simulink model "test_model_ver1"  (R2018a)
settings: Solver=FixedStepAuto  StartTime=0.0  StopTime=789  FixedStep=1  RelTol=1e-3
PreLoadFcn:
  | load '../simulink/model_specs/LSTM/n_LSTM_units.mat'
  | load '../simulink/model_specs/LSTM/T.mat'
  | load '../simulink/model_specs/LSTM/data_input_weights.mat'
  | load '../simulink/model_specs/LSTM/h_weights.mat'
  | load '../simulink/model_specs/LSTM/gate_bias.mat'
  | load '../simulink/model_specs/MLP/weight1.mat'
  | load '../simulink/model_specs/MLP/bias1.mat'
  | load '../simulink/model_specs/MLP/weight2.mat'
  | load '../simulink/model_specs/MLP/bias2.mat'
PostLoadFcn:
  | load 'model_specs/LSTM/n_LSTM_units.mat'
  | load 'model_specs/LSTM/T.mat'
  | load 'model_specs/LSTM/data_input_weights.mat'
  | load 'model_specs/LSTM/h_weights.mat'
  | load 'model_specs/LSTM/gate_bias.mat'
  | load 'model_specs/MLP/weight1.mat'
  | load 'model_specs/MLP/bias1.mat'
  | load 'model_specs/MLP/weight2.mat'
  | load 'model_specs/MLP/bias2.mat'
undefined symbols (not defined in the file): bias1, bias2, data_input_weights, gate_bias, h_weights, n_LSTM_units, weight1, weight2
settings Model: Creator=tongl  LastModifiedBy=tongl

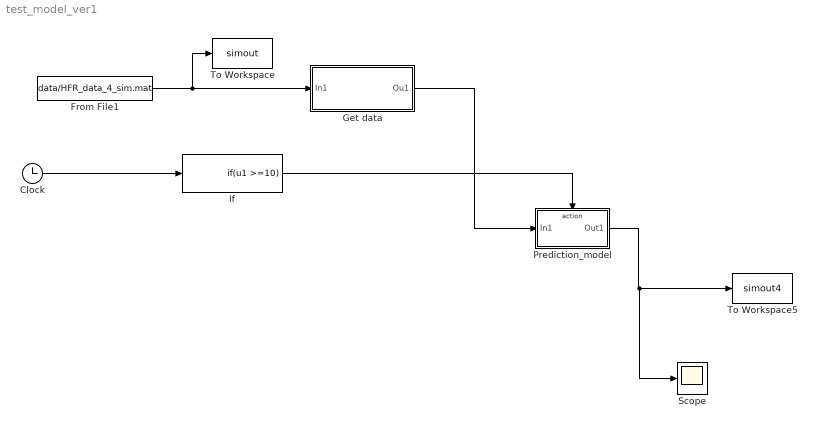
== system test_model_ver1 ==
  Clock : Clock
  From File1 : FromFile  FileName=data/HFR_data_4_sim.mat  OutDataTypeStr=double  SampleTime=1  ExtrapolationBeforeFirstDataPoint=Hold first value
  Get data : Subsystem  Tag=Get_Data
  If : If  IfExpression=u1 >=10  ShowElse=off
  "Prediction_model " : Subsystem  TreatAsAtomicUnit=on
  Scope : Scope
  To Workspace : ToWorkspace  VariableName=simout  SaveFormat=Timeseries  SampleTime=-1
  To Workspace5 : ToWorkspace  VariableName=simout4  SaveFormat=Timeseries  SampleTime=-1
  wires:
  Clock/1 -> If/1
  If/1 -> "Prediction_model "/Action
  "Prediction_model "/1(Out1) -> Scope/1, To Workspace5/1
  From File1/1 -> To Workspace/1, Get data/1(In1)
  Get data/1(Ou1) -> "Prediction_model "/1(In1)

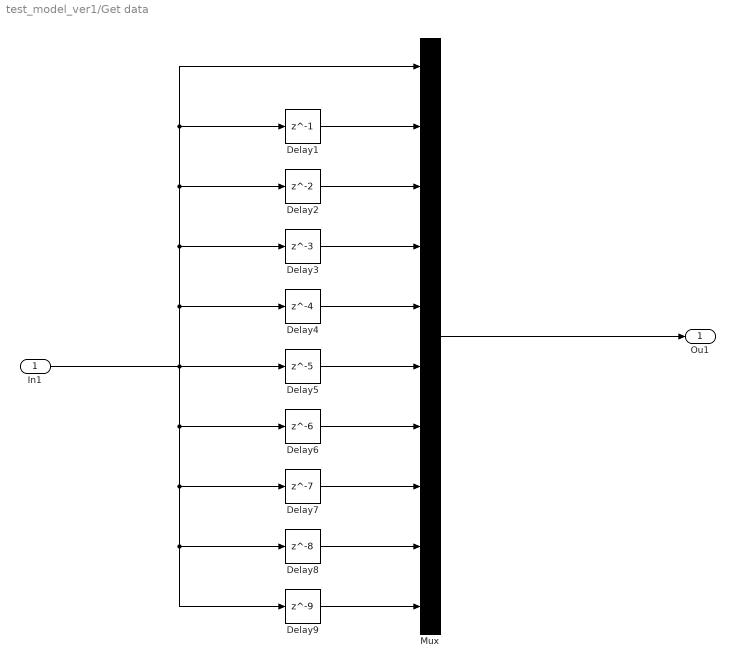
== system test_model_ver1/Get data ==
  In1 : Inport
  Delay1 : Delay  DelayLength=1  InitialCondition=0
  Delay2 : Delay  InitialCondition=0
  Delay3 : Delay  DelayLength=3  InitialCondition=0
  Delay4 : Delay  DelayLength=4  InitialCondition=0
  Delay5 : Delay  DelayLength=5  InitialCondition=0
  Delay6 : Delay  DelayLength=6  InitialCondition=0
  Delay7 : Delay  DelayLength=7  InitialCondition=0
  Delay8 : Delay  DelayLength=8  InitialCondition=0
  Delay9 : Delay  DelayLength=9  InitialCondition=0
  Mux : Mux  Inputs=10
  Ou1 : Outport
  wires:
  Delay2/1 -> Mux/3
  Delay3/1 -> Mux/4
  Delay8/1 -> Mux/9
  Delay7/1 -> Mux/8
  Delay6/1 -> Mux/7
  Delay4/1 -> Mux/5
  Delay1/1 -> Mux/2
  Delay9/1 -> Mux/10
  Delay5/1 -> Mux/6
  Mux/1 -> Ou1/1
  In1/1 -> Delay7/1, Delay9/1, Delay8/1, Delay6/1, Delay5/1, Delay4/1, Delay3/1, Delay2/1, Mux/1, Delay1/1

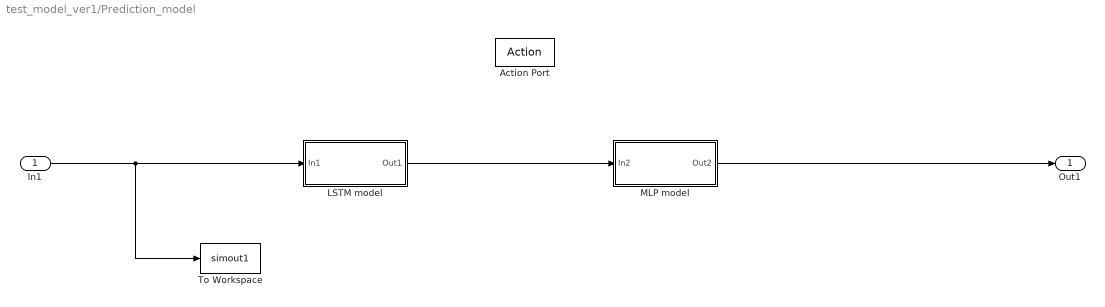
== system test_model_ver1/Prediction_model  ==
  In1 : Inport
  Action Port : ActionPort  ActionType=then
  LSTM model : Subsystem  TreatAsAtomicUnit=on
  MLP model : Subsystem
  To Workspace : ToWorkspace  VariableName=simout1  SaveFormat=Timeseries  SampleTime=-1
  Out1 : Outport
  wires:
  In1/1 -> To Workspace/1, LSTM model/1(In1)
  LSTM model/1(Out1) -> MLP model/1(In2)
  MLP model/1(Out2) -> Out1/1

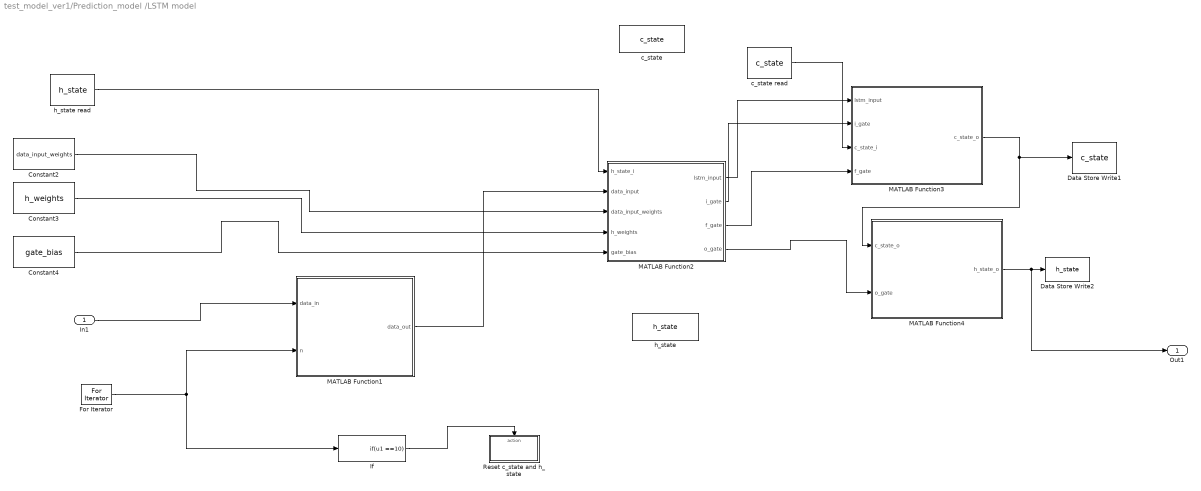
== system test_model_ver1/Prediction_model /LSTM model ==
  In1 : Inport
  Constant2 : Constant  Value=data_input_weights
  Constant3 : Constant  Value=h_weights
  Constant4 : Constant  Value=gate_bias
  Data Store Write1 : DataStoreWrite  DataStoreName=c_state
  Data Store Write2 : DataStoreWrite  DataStoreName=h_state
  For Iterator : ForIterator  IterationLimit=10
  If : If  IfExpression=u1 ==10  ShowElse=off
  MATLAB Function1 : MATLAB Function  TreatAsAtomicUnit=on
  MATLAB Function2 : MATLAB Function  TreatAsAtomicUnit=on
  MATLAB Function3 : MATLAB Function  TreatAsAtomicUnit=on
  MATLAB Function4 : MATLAB Function  TreatAsAtomicUnit=on
  Reset c_state and h_state : Subsystem  TreatAsAtomicUnit=on
  c_state : DataStoreMemory  DataStoreName=c_state  ReadBeforeWriteMsg=warning  WriteAfterWriteMsg=warning  WriteAfterReadMsg=warning  InitialValue=zeros(256,1)  ShowAdditionalParam=off  OutDataTypeStr=single  Dimensions=[n_LSTM_units,1]
  c_state read : DataStoreRead  DataStoreName=c_state
  h_state : DataStoreMemory  DataStoreName=h_state  ReadBeforeWriteMsg=warning  WriteAfterWriteMsg=warning  WriteAfterReadMsg=warning  InitialValue=zeros(256,1)  ShowAdditionalParam=off  OutDataTypeStr=single  Dimensions=[n_LSTM_units,1]
  h_state read : DataStoreRead  DataStoreName=h_state
  Out1 : Outport
  wires:
  h_state read/1 -> MATLAB Function2/1(h_state_i)
  MATLAB Function4/1(h_state_o) -> Out1/1, Data Store Write2/1
  Constant3/1 -> MATLAB Function2/4(h_weights)
  MATLAB Function3/1(c_state_o) -> MATLAB Function4/1(c_state_o), Data Store Write1/1
  MATLAB Function2/4(o_gate) -> MATLAB Function4/2(o_gate)
  MATLAB Function2/1(lstm_input) -> MATLAB Function3/1(lstm_input)
  Constant2/1 -> MATLAB Function2/3(data_input_weights)
  c_state read/1 -> MATLAB Function3/3(c_state_i)
  MATLAB Function2/2(i_gate) -> MATLAB Function3/2(i_gate)
  MATLAB Function2/3(f_gate) -> MATLAB Function3/4(f_gate)
  Constant4/1 -> MATLAB Function2/5(gate_bias)
  In1/1 -> MATLAB Function1/1(data_in)
  For Iterator/1 -> If/1, MATLAB Function1/2(n)
  MATLAB Function1/1(data_out) -> MATLAB Function2/2(data_input)
  If/1 -> Reset c_state and h_state/Action

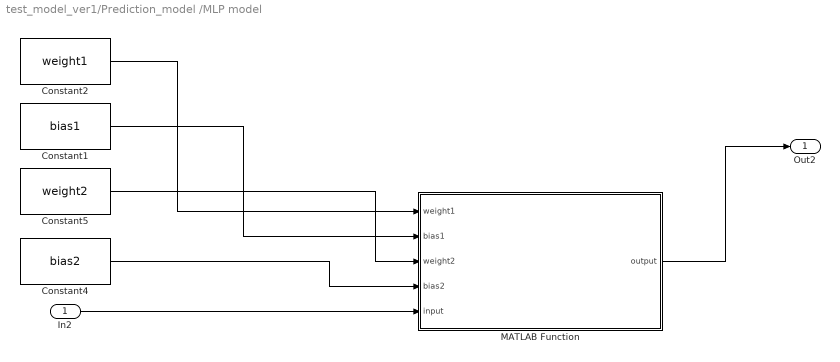
== system test_model_ver1/Prediction_model /MLP model ==
  In2 : Inport
  Constant1 : Constant  Value=bias1
  Constant2 : Constant  Value=weight1
  Constant4 : Constant  Value=bias2
  Constant5 : Constant  Value=weight2
  MATLAB Function : MATLAB Function  TreatAsAtomicUnit=on
  Out2 : Outport  OutDataTypeStr=single
  wires:
  In2/1 -> MATLAB Function/5(input)
  Constant1/1 -> MATLAB Function/2(bias1)
  MATLAB Function/1(output) -> Out2/1
  Constant4/1 -> MATLAB Function/4(bias2)
  Constant5/1 -> MATLAB Function/3(weight2)
  Constant2/1 -> MATLAB Function/1(weight1)

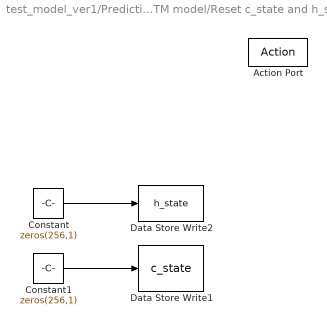
== system test_model_ver1/Prediction_model /LSTM model/Reset c_state and h_state ==
  Action Port : ActionPort  ActionType=then
  Constant : Constant  Value=zeros(256,1)  OutDataTypeStr=single
  Constant1 : Constant  Value=zeros(256,1)  OutDataTypeStr=single
  Data Store Write1 : DataStoreWrite  DataStoreName=c_state
  Data Store Write2 : DataStoreWrite  DataStoreName=h_state
  wires:
  Constant/1 -> Data Store Write2/1
  Constant1/1 -> Data Store Write1/1

== matlab function test_model_ver1/Prediction_model /LSTM model/MATLAB Function2 ==
  data: h_state_i input; data_input input; data_input_weights input; h_weights input; gate_bias input; lstm_input output size=[n_LSTM_units,1] [-1000..1000]; i_gate output; f_gate output; o_gate output
function [lstm_input,i_gate,f_gate,o_gate]=compute_gates(h_state_i,data_input,data_input_weights,h_weights,gate_bias)
%%%% this function computes the gate mechanism of lstm 
%%%% data_input_weights: weights for data inputs (W_input + W_input_gate+W_forget_gate+W_output_gate) * sizeof data_input 
%%%% h_input_weights: weights for previous h (W_input + W_input_gate+W_forget_gate+W_output_gate) * sizeof h 
%%%% gate_bias: [(b_input + b_input_gate+ b_forget_gate + b_output_gate)]*1

n_LSTM_units=256; %%%% LSTM hidden units 

%%%% Initialization %%%%
combine=zeros(4*n_LSTM_units,1,'single');
i_gate=zeros(n_LSTM_units,1,'single');
f_gate=zeros(n_LSTM_units,1,'single');
lstm_input=zeros(n_LSTM_units,1,'single');
o_gate=ones(n_LSTM_units,1,'single');

% data_input=single(data_input(i*feature+1:(i+1)*feature));

combine=data_input_weights*data_input+h_weights*h_state_i+gate_bias; %%%4n_h*1 %%% compute the inputs before sigmoid
i_gate=sigmoid(combine(1:n_LSTM_units,1)); %%% n_h*1
f_gate=sigmoid(combine(n_LSTM_units+1:2*n_LSTM_units,1)); %%% n_h*1
lstm_input=tanh(combine(2*n_LSTM_units+1:3*n_LSTM_units,1)); %%% n_h*1
o_gate=sigmoid(combine(3*n_LSTM_units+1:4*n_LSTM_units,1)); %%% n_h*1
end

function output=my_tanh(input) %%% not sure if this can be implemented 
a=1-exp(-2*input); %%% use negative coeff to avoid overflow
b=1+exp(-2*input);  
output=a./b;
end

function output=sigmoid(input) %%% not sure if this can be implemented 
%%% help function: sigmoid 
a=1; 
b=exp(-input)+1;  %%% use negative coeff to avoid overflow
output=a./b;
% if sum(sum(isnan(output)))~=0
%      a=1
% end 
end

== matlab function test_model_ver1/Prediction_model /LSTM model/MATLAB Function3 ==
  data: lstm_input input; i_gate input; c_state_i input; f_gate input; c_state_o output
function c_state_o=compute_cell_state(lstm_input,i_gate,c_state_i,f_gate)
%%%% compute lstm cell states


current_update=lstm_input.*i_gate;
previous_correction=c_state_i.*f_gate; %%% n_h *1 
c_state_o=current_update+previous_correction;  %%% n_h*1
end

== matlab function test_model_ver1/Prediction_model /LSTM model/MATLAB Function1 ==
  data: data_in input; n input; data_out output [-10000..10000]
function data_out =organize_data(data_in,n)
%%%% THis function get feature_size*1 data input from (feature_size*look_back_step,1) data 
%%%% data_in: data for LSTM input (feature_size*look_back_step,1), last feature_size*1 data is the most recent sensor readingViswanathan 
%%%% n: iteration number, same as LSTM look back length  

T=10; %%% Total look back length 
feature=12; %%% feature size 
%%%% extract data %%%%%
data_out=zeros(feature,1,'single'); 
data_out=single(data_in((T-n)*feature+1:(T-n+1)*feature));
data_out=reshape(data_out,feature,1);
end

== matlab function test_model_ver1/Prediction_model /LSTM model/MATLAB Function4 ==
  data: c_state_o input; o_gate input; h_state_o output
function h_state_o=compute_output(c_state_o,o_gate)
%%% compute lstm output 
h_state_o=my_tanh(c_state_o).*o_gate; %%% n_h*1
end 

function output=my_tanh(input) %%% not sure if this can be implemented 
a=1-exp(-2*input); %%% use negative coeff to avoid overflow
b=1+exp(-2*input);  
output=a./b;
end

== matlab function test_model_ver1/Prediction_model /MLP model/MATLAB Function ==
  data: weight1 input; output output; bias1 input; weight2 input; bias2 input; input input
function output= MLP_forward(weight1,bias1,weight2,bias2,input)
%% input: feature_size*1

%%%: need to combine two dense layers or add non-avtivation in between, will change in future

% weight1=model_specs.weight1;
% bias1=model_specs.bias1;
% weight2=model_specs.weight2;
% bias2=model_specs.bias2;
 
output_1=single(zeros(256,1)); 
relu1=single(zeros(1,256));
output=single(zeros(1,1));  
weight2=reshape(weight2,1,256); %%% reshape for the shape "1"*256 

output_1=dense_layer(input,weight1,bias1); 
relu_1=ReLU_layer(output_1); 

output=dense_layer(relu_1,weight2,bias2);
end

function result=dense_layer(input,weight,bias)
%%% fully connected layer 
result=weight*input+bias;
end 

function result = ReLU_layer(input) 
result=(input>0).*input; %%% not sure if can be complied 
end
